simulink model "atrias_on_boom"  (R2018b)
settings: Solver=ode15s  StartTime=0.0  StopTime=inf  FixedStep=sample_time  MaxStep=1e-2  RelTol=1e-3
InitFcn:
  | addpath('../common/')
  | colors
  | simulation_params
  | mechanical_params
StartFcn:
  | clc
  | tic
StopFcn:
  | stopscript
values from neighbouring files (symbols this model uses):
  sample_time = 1/sample_freq    (= 0.001)    [simulation_params.m]
undefined symbols (not defined in the file or in its folder): Force_Control, rad, s, sgn, sm, t_friction, X, Y, Z
libraries: sm_lib x205, nesl_utility x123, simulink x49, fl_lib x16, mblibv1 x4, simulink_extras x2, powerlib_meascontrol x1
(part 8 of 8)

== system atrias_on_boom/Mechanical System Layer/R Leg/Thigh SEA/Rotor and Gearing ==
  Rotor Torque [Nm] : Inport
  Spring Torque [Nm] : Inport  Port=2
  Aligned Gear Constraint : sm_lib/Gears and Couplings/Gears/Common Gear Constraint  GearType=External  SpecificationType=CenterDistanceRatio  CenterDistance=(sm.r_rotor+sm.r_virtual_gear)/2  CenterDistanceUnits=m  GearRatio=1  BaseGearRadius=1  BaseGearRadiusUnits=m  FollGearRadius=1  FollGearRadiusUnits=m  AssemblyGearRotation=Free
      settings: SourceProductName=Simscape Multibody  SourceProductBaseCode=MS
  External Force and Torque : sm_lib/Forces and Torques/External Force and Torque  ForceResolutionFrame=AttachedFrame  EnableForceX=off  EnableForceY=off  EnableForceZ=off  EnableForce=off  TorqueResolutionFrame=AttachedFrame  EnableTorqueX=off  EnableTorqueY=off  EnableTorqueZ=on  EnableTorque=off
  Gear Offset : sm_lib/Frames and Transforms/Rigid Transform  TranslationMethod=Cartesian  TranslationStandardOffset=0  TranslationLengthUnit=m  TranslationStandardAxis=+Z  TranslationCartesianOffset=[(sm.r_rotor+sm.r_virtual_gear) 0 0]  TranslationROffset=0  TranslationROffsetUnits=m  TranslationZOffset=0  TranslationZOffsetUnits=m  TranslationThetaOffset=0  TranslationThetaOffsetUnits=deg  RotationMethod=None  RotationAngleUnits=deg  RotationStandardAxis=+Z  RotationAngle=0  RotationArbitraryAxis=[0 0 1]  FollAlignAxisA=+X  BaseAlignAxisA=+Y  FollAlignAxisB=+Y  BaseAlignAxisB=+Z  RotationSequenceAxes=FollowerAxes  RotationSequence=XYX  RotationSequenceAngles=[0 0 0]  RotationSequenceAnglesUnits=deg  RotationMatrix=[1 0 0; 0 1 0; 0 0 1]
  Idler Gear : sm_lib/Body Elements/Solid  InertiaType=Custom  Mass=sm.m_virtual_gear  MassUnits=kg  CenterOfMass=[0 0 0]  CenterOfMassUnits=m  MomentsOfInertia=sm.i_virtual_gear  MomentsOfInertiaUnits=kg*m^2  ProductsOfInertia=[0 0 0]  ProductsOfInertiaUnits=kg*m^2  BasedOnType=Density  Density=1000  DensityUnits=kg/(m^3)  DoExposeReferenceFrame=on  SerializedFrames=<Frames/>  GraphicType=None  MarkerShape=Sphere  MarkerSize=10  MarkerSizeUnits=m  GraphicVisPropType=SimpleVisualProperties  GraphicDiffuseColor=[1.0 0.2 0.2]  GraphicSpecularColor=[0.5 0.5 0.5 1.0]  GraphicAmbientColor=[0.15 0.15 0.15 1.0]  GraphicEmissiveColor=[0.0 0.0 0.0 1.0]  GraphicShininess=75  GraphicOpacity=1.0  GeometryShape=Cylinder  RectangleSize=[1 1]  RectangleSizeUnits=m  BrickDimensions=[1 1 1]  BrickDimensionUnits=m  CylinderRadius=sm.r_virtual_gear  CylinderRadiusUnits=m  CylinderLength=0.01  CylinderLengthUnits=m  SphereRadius=1  SphereRadiusUnits=m  EllipsoidRadii=[1 1 1]  EllipsoidRadiiUnits=m  ExtrusionCrossSection=[1 1; -1 1; -1 -1; 1 -1]  ExtrusionCrossSectionUnits=m  ExtrusionLength=.2  ExtrusionLengthUnits=m  PolygonNumSides=3  PolygonOuterRadius=.3  PolygonOuterRadiusUnits=m  ExtGeomFileType=STL  ExtGeomFileUnits=m  RevolutionCrossSection=[1 1; 1 -1; 2 -1; 2 1]  RevolutionCrossSectionUnits=m  RevolutionExtent=Full  RevolutionAngle=180  RevolutionAngleUnits=deg
  Idler Gear Constraint : sm_lib/Gears and Couplings/Gears/Common Gear Constraint  GearType=External  SpecificationType=CenterDistanceRatio  CenterDistance=(sm.r_rotor+sm.r_virtual_gear)/2  CenterDistanceUnits=m  GearRatio=1.0  BaseGearRadius=1  BaseGearRadiusUnits=m  FollGearRadius=1  FollGearRadiusUnits=m  AssemblyGearRotation=Free
      settings: SourceProductName=Simscape Multibody  SourceProductBaseCode=MS
  Idler Offset : sm_lib/Frames and Transforms/Rigid Transform  TranslationMethod=Cartesian  TranslationStandardOffset=0  TranslationLengthUnit=m  TranslationStandardAxis=+Z  TranslationCartesianOffset=[(sm.r_rotor+sm.r_virtual_gear)/2 0 0]  TranslationROffset=0  TranslationROffsetUnits=m  TranslationZOffset=0  TranslationZOffsetUnits=m  TranslationThetaOffset=0  TranslationThetaOffsetUnits=deg  RotationMethod=None  RotationAngleUnits=deg  RotationStandardAxis=+Z  RotationAngle=0  RotationArbitraryAxis=[0 0 1]  FollAlignAxisA=+X  BaseAlignAxisA=+Y  FollAlignAxisB=+Y  BaseAlignAxisB=+Z  RotationSequenceAxes=FollowerAxes  RotationSequence=XYX  RotationSequenceAngles=[0 0 0]  RotationSequenceAnglesUnits=deg  RotationMatrix=[1 0 0; 0 1 0; 0 0 1]
  Mechanical Rotational Reference : fl_lib/Mechanical/Rotational Elements/Mechanical Rotational Reference
  Opposite : Gain  Gain=-1
  Output Gear Joint : sm_lib/Joints/Revolute Joint  SenseConstraintForce=off  SenseConstraintForceX=off  SenseConstraintForceY=off  SenseConstraintForceZ=off  SenseConstraintTorque=off  SenseConstraintTorqueX=off  SenseConstraintTorqueY=off  SenseConstraintTorqueZ=off  SenseTotalForce=off  SenseTotalForceX=off  SenseTotalForceY=off  SenseTotalForceZ=off  SenseTotalTorque=off  SenseTotalTorqueX=off  SenseTotalTorqueY=off  SenseTotalTorqueZ=off  CompositeWrenchDir=FollowerOnBase  CompositeWrenchFrame=BaseFrame  EquilibriumPosition=0  EquilibriumPositionUnits=deg  SpringStiffness=0  SpringStiffnessUnits=N*m/deg  DampingCoefficient=0  DampingCoefficientUnits=N*m/(deg/s)  TorqueActuationMode=NoTorque  MotionActuationMode=ComputedMotion  SensePosition=on  SenseVelocity=on  SenseAcceleration=off  SenseTorqueForce=off  PositionTargetSpecify=off  PositionTargetPriority=High  PositionTargetValue=0  PositionTargetValueUnits=deg  VelocityTargetSpecify=off  VelocityTargetPriority=High  VelocityTargetValue=0  VelocityTargetValueUnits=deg/s
  Output Gear : sm_lib/Body Elements/Solid  InertiaType=Custom  Mass=sm.m_output_gear  MassUnits=kg  CenterOfMass=[0 0 0]  CenterOfMassUnits=m  MomentsOfInertia=sm.i_output_gear  MomentsOfInertiaUnits=kg*m^2  ProductsOfInertia=[0 0 0]  ProductsOfInertiaUnits=kg*m^2  BasedOnType=Density  Density=1000  DensityUnits=kg/(m^3)  DoExposeReferenceFrame=on  SerializedFrames=<Frames/>  GraphicType=None  MarkerShape=Sphere  MarkerSize=10  MarkerSizeUnits=m  GraphicVisPropType=SimpleVisualProperties  GraphicDiffuseColor=[1.0 0.2 0.0]  GraphicSpecularColor=[0.5 0.5 0.5 1.0]  GraphicAmbientColor=[0.15 0.15 0.15 1.0]  GraphicEmissiveColor=[0.0 0.0 0.0 1.0]  GraphicShininess=75  GraphicOpacity=1.0  GeometryShape=Cylinder  RectangleSize=[1 1]  RectangleSizeUnits=m  BrickDimensions=[1 1 1]  BrickDimensionUnits=m  CylinderRadius=0.03  CylinderRadiusUnits=m  CylinderLength=0.01  CylinderLengthUnits=m  SphereRadius=1  SphereRadiusUnits=m  EllipsoidRadii=[1 1 1]  EllipsoidRadiiUnits=m  ExtrusionCrossSection=[1 1; -1 1; -1 -1; 1 -1]  ExtrusionCrossSectionUnits=m  ExtrusionLength=1  ExtrusionLengthUnits=m  PolygonNumSides=3  PolygonOuterRadius=1  PolygonOuterRadiusUnits=m  ExtGeomFileType=STL  ExtGeomFileUnits=m  RevolutionCrossSection=[1 1; 1 -1; 2 -1; 2 1]  RevolutionCrossSectionUnits=m  RevolutionExtent=Full  RevolutionAngle=180  RevolutionAngleUnits=deg
  PS-Simulink Converter{,1..3} (4 alike) : nesl_utility/PS-Simulink Converter  PhysicalDomain=network_engine_domain  SubClassName=ps_output  LeftPortType=input  RightPortType=output  PseudoPeriodic=off  Frequencies=[]  Unit=1  AffineConversion=off
  Rotational Simscape Intf : Subsystem
  Rotational Friction : fl_lib/Mechanical/Rotational Elements/Rotational Friction  brkwy_trq=sm.breakaway_friction(2)/sm.N N*m  brkwy_vel=exp(-( (sm.friction_linear_zone(2)*sm.N) * 1 * (10) * 1 + 1/2) ) * ( (sm.friction_linear_zone(2)*sm.N) * 1 / 2 + 1 / ( (10) * 1) ) rad/s  Col_trq=sm.coulomb_friction(2)/sm.N N*m  visc_coef=sm.viscous_friction(2)/sm.N N*m/(rad/s)  w_specify=off  w_priority=High  w=0 rad/s  w_nominal_specify=off  w_nominal_unit=rad/s  w_nominal_value=1  t_specify=off  t_priority=High  t=0 N*m  t_nominal_specify=off  t_nominal_unit=N*m  t_nominal_value=1
      settings: SourceProductName=Simscape
  Rotor + Base Gear : sm_lib/Body Elements/Solid  InertiaType=Custom  Mass=sm.m_rotor  MassUnits=kg  CenterOfMass=[0 0 0]  CenterOfMassUnits=m  MomentsOfInertia=sm.i_rotor_moments  MomentsOfInertiaUnits=kg*m^2  ProductsOfInertia=[0 0 0]  ProductsOfInertiaUnits=kg*m^2  BasedOnType=Density  Density=1000  DensityUnits=kg/(m^3)  DoExposeReferenceFrame=on  SerializedFrames=<Frames/>  GraphicType=None  MarkerShape=Sphere  MarkerSize=10  MarkerSizeUnits=m  GraphicVisPropType=AdvancedVisualProperties  GraphicDiffuseColor=[0.5 0.5 0.5]  GraphicSpecularColor=[0.5 0.5 0.5 1.0]  GraphicAmbientColor=[0.15 0.15 0.15 1.0]  GraphicEmissiveColor=[0.0 0.0 0.0 1.0]  GraphicShininess=10  GraphicOpacity=1.0  GeometryShape=Cylinder  RectangleSize=[1 1]  RectangleSizeUnits=m  BrickDimensions=[1 1 1]  BrickDimensionUnits=m  CylinderRadius=0.01  CylinderRadiusUnits=m  CylinderLength=0.01  CylinderLengthUnits=m  SphereRadius=1  SphereRadiusUnits=m  EllipsoidRadii=[1 1 1]  EllipsoidRadiiUnits=m  ExtrusionCrossSection=[1 1; -1 1; -1 -1; 1 -1]  ExtrusionCrossSectionUnits=m  ExtrusionLength=0.4  ExtrusionLengthUnits=m  PolygonNumSides=3  PolygonOuterRadius=0.2  PolygonOuterRadiusUnits=m  ExtGeomFileType=STL  ExtGeomFileUnits=m  RevolutionCrossSection=[1 1; 1 -1; 2 -1; 2 1]  RevolutionCrossSectionUnits=m  RevolutionExtent=Full  RevolutionAngle=180  RevolutionAngleUnits=deg
  Rotor Joint : sm_lib/Joints/Revolute Joint  SenseConstraintForce=off  SenseConstraintForceX=off  SenseConstraintForceY=off  SenseConstraintForceZ=off  SenseConstraintTorque=off  SenseConstraintTorqueX=off  SenseConstraintTorqueY=off  SenseConstraintTorqueZ=off  SenseTotalForce=off  SenseTotalForceX=off  SenseTotalForceY=off  SenseTotalForceZ=off  SenseTotalTorque=off  SenseTotalTorqueX=off  SenseTotalTorqueY=off  SenseTotalTorqueZ=off  CompositeWrenchDir=FollowerOnBase  CompositeWrenchFrame=BaseFrame  EquilibriumPosition=0  EquilibriumPositionUnits=deg  SpringStiffness=0  SpringStiffnessUnits=N*m/deg  DampingCoefficient=0  DampingCoefficientUnits=N*m/(deg/s)  TorqueActuationMode=InputTorque  MotionActuationMode=ComputedMotion  SensePosition=off  SenseVelocity=on  SenseAcceleration=off  SenseTorqueForce=off  PositionTargetSpecify=off  PositionTargetPriority=High  PositionTargetValue=0  PositionTargetValueUnits=deg  VelocityTargetSpecify=off  VelocityTargetPriority=High  VelocityTargetValue=0  VelocityTargetValueUnits=deg/s
  Simulink-PS Converter : nesl_utility/Simulink-PS Converter  PhysicalDomain=network_engine_domain  SubClassName=ps_input  LeftPortType=input  RightPortType=output  PseudoPeriodic=off  Frequencies=[]  NoiseDistribution=none  NoiseParameters=[]  Unit=1  AffineConversion=off  FilteringAndDerivatives=zero  SimscapeFilterOrder=1  InputFilterTimeConstant=0.001  UdotUserProvided=1
  Simulink-PS Converter1 : nesl_utility/Simulink-PS Converter  PhysicalDomain=network_engine_domain  SubClassName=ps_input  LeftPortType=input  RightPortType=output  PseudoPeriodic=off  Frequencies=[]  NoiseDistribution=none  NoiseParameters=[]  Unit=1  AffineConversion=off  FilteringAndDerivatives=zero  SimscapeFilterOrder=1  InputFilterTimeConstant=0.001  UdotUserProvided=1
  Sum : Sum  Inputs=|++
  Virtual Gear Joint : sm_lib/Joints/Revolute Joint  SenseConstraintForce=off  SenseConstraintForceX=off  SenseConstraintForceY=off  SenseConstraintForceZ=off  SenseConstraintTorque=off  SenseConstraintTorqueX=off  SenseConstraintTorqueY=off  SenseConstraintTorqueZ=off  SenseTotalForce=off  SenseTotalForceX=off  SenseTotalForceY=off  SenseTotalForceZ=off  SenseTotalTorque=off  SenseTotalTorqueX=off  SenseTotalTorqueY=off  SenseTotalTorqueZ=off  CompositeWrenchDir=FollowerOnBase  CompositeWrenchFrame=BaseFrame  EquilibriumPosition=0  EquilibriumPositionUnits=deg  SpringStiffness=0  SpringStiffnessUnits=N*m/deg  DampingCoefficient=0  DampingCoefficientUnits=N*m/(deg/s)  TorqueActuationMode=NoTorque  MotionActuationMode=ComputedMotion  SensePosition=off  SenseVelocity=off  SenseAcceleration=off  SenseTorqueForce=off  PositionTargetSpecify=off  PositionTargetPriority=High  PositionTargetValue=0  PositionTargetValueUnits=deg  VelocityTargetSpecify=off  VelocityTargetPriority=High  VelocityTargetValue=0  VelocityTargetValueUnits=deg/s
  Virtual Follower Gear : sm_lib/Body Elements/Solid  InertiaType=Custom  Mass=sm.m_virtual_gear  MassUnits=kg  CenterOfMass=[0 0 0]  CenterOfMassUnits=m  MomentsOfInertia=sm.i_virtual_gear  MomentsOfInertiaUnits=kg*m^2  ProductsOfInertia=[0 0 0]  ProductsOfInertiaUnits=kg*m^2  BasedOnType=Density  Density=1000  DensityUnits=kg/(m^3)  DoExposeReferenceFrame=on  SerializedFrames=<Frames/>  GraphicType=None  MarkerShape=Sphere  MarkerSize=10  MarkerSizeUnits=m  GraphicVisPropType=SimpleVisualProperties  GraphicDiffuseColor=[1.0 0.2 0.2]  GraphicSpecularColor=[0.5 0.5 0.5 1.0]  GraphicAmbientColor=[0.15 0.15 0.15 1.0]  GraphicEmissiveColor=[0.0 0.0 0.0 1.0]  GraphicShininess=75  GraphicOpacity=1.0  GeometryShape=Cylinder  RectangleSize=[1 1]  RectangleSizeUnits=m  BrickDimensions=[1 1 1]  BrickDimensionUnits=m  CylinderRadius=sm.r_virtual_gear  CylinderRadiusUnits=m  CylinderLength=0.01  CylinderLengthUnits=m  SphereRadius=1  SphereRadiusUnits=m  EllipsoidRadii=[1 1 1]  EllipsoidRadiiUnits=m  ExtrusionCrossSection=[1 1; -1 1; -1 -1; 1 -1]  ExtrusionCrossSectionUnits=m  ExtrusionLength=.2  ExtrusionLengthUnits=m  PolygonNumSides=3  PolygonOuterRadius=.3  PolygonOuterRadiusUnits=m  ExtGeomFileType=STL  ExtGeomFileUnits=m  RevolutionCrossSection=[1 1; 1 -1; 2 -1; 2 1]  RevolutionCrossSectionUnits=m  RevolutionExtent=Full  RevolutionAngle=180  RevolutionAngleUnits=deg
  Virtual Gear Constraint : sm_lib/Gears and Couplings/Gears/Common Gear Constraint  GearType=External  SpecificationType=PitchCircleRadii  CenterDistance=20.0  CenterDistanceUnits=cm  GearRatio=1.0  BaseGearRadius=sm.r_rotor  BaseGearRadiusUnits=m  FollGearRadius=sm.r_virtual_gear  FollGearRadiusUnits=m  AssemblyGearRotation=Free
      settings: SourceProductName=Simscape Multibody  SourceProductBaseCode=MS
  Virtual Idler : sm_lib/Joints/Revolute Joint  SenseConstraintForce=off  SenseConstraintForceX=off  SenseConstraintForceY=off  SenseConstraintForceZ=off  SenseConstraintTorque=off  SenseConstraintTorqueX=off  SenseConstraintTorqueY=off  SenseConstraintTorqueZ=off  SenseTotalForce=off  SenseTotalForceX=off  SenseTotalForceY=off  SenseTotalForceZ=off  SenseTotalTorque=off  SenseTotalTorqueX=off  SenseTotalTorqueY=off  SenseTotalTorqueZ=off  CompositeWrenchDir=FollowerOnBase  CompositeWrenchFrame=BaseFrame  EquilibriumPosition=0  EquilibriumPositionUnits=deg  SpringStiffness=0  SpringStiffnessUnits=N*m/deg  DampingCoefficient=0  DampingCoefficientUnits=N*m/(deg/s)  TorqueActuationMode=NoTorque  MotionActuationMode=ComputedMotion  SensePosition=off  SenseVelocity=off  SenseAcceleration=off  SenseTorqueForce=off  PositionTargetSpecify=off  PositionTargetPriority=High  PositionTargetValue=0  PositionTargetValueUnits=deg  VelocityTargetSpecify=off  VelocityTargetPriority=High  VelocityTargetValue=0  VelocityTargetValueUnits=deg/s
  Rotor Conn : PMIOPort  Side=Left
  Gearhead Position [rad] : Outport
  Gearhead Velocity [rad/s] : Outport  Port=2
  Rotor Velocity [rad/s] : Outport  Port=3
  wires:
  PS-Simulink Converter1/1 -> Gearhead Position [rad]/1
  Rotor Torque [Nm]/1 -> Sum/1
  PS-Simulink Converter2/1 -> Gearhead Velocity [rad/s]/1
  PS-Simulink Converter3/1 -> Rotor Velocity [rad/s]/1
  Spring Torque [Nm]/1 -> Opposite/1
  Opposite/1 -> Simulink-PS Converter1/1
  Sum/1 -> Simulink-PS Converter/1
  PS-Simulink Converter/1 -> Sum/2
  connections:
  Virtual Gear Joint/RConn1 -- Virtual Follower Gear/RConn1 -- Virtual Gear Constraint/RConn1 -- Idler Gear Constraint/LConn1
  External Force and Torque/RConn1 -- Output Gear/RConn1 -- Aligned Gear Constraint/RConn1 -- Output Gear Joint/RConn1
  Gear Offset/RConn1 -- Virtual Gear Joint/LConn1
  Gear Offset/LConn1 -- Rotor Joint/LConn1 -- Rotor Conn/RConn1 -- Output Gear Joint/LConn1 -- Idler Offset/LConn1
  Rotor Joint/RConn1 -- Virtual Gear Constraint/LConn1 -- Rotor + Base Gear/RConn1
  Simulink-PS Converter/RConn1 -- Rotor Joint/LConn2
  PS-Simulink Converter2/LConn1 -- Output Gear Joint/RConn3
  PS-Simulink Converter1/LConn1 -- Output Gear Joint/RConn2
  PS-Simulink Converter3/LConn1 -- Rotational Simscape Intf/LConn1 -- Rotor Joint/RConn2
  Simulink-PS Converter1/RConn1 -- External Force and Torque/LConn1
  Idler Gear Constraint/RConn1 -- Virtual Idler/RConn1 -- Idler Gear/RConn1 -- Aligned Gear Constraint/LConn1
  Idler Offset/RConn1 -- Virtual Idler/LConn1
  PS-Simulink Converter/LConn1 -- Rotational Simscape Intf/RConn1
  Rotational Friction/RConn1 -- Mechanical Rotational Reference/LConn1 -- Rotational Simscape Intf/RConn2
  Rotational Friction/LConn1 -- Rotational Simscape Intf/LConn2

== system atrias_on_boom/Mechanical System Layer/Right Hip Roll Joint/Mechanical Limits /Enabled Subsystem ==
  Col_Flags : Inport
  Enable : EnablePort  StatesWhenEnabling=reset  ZeroCross=off
  To Workspace : ToWorkspace  VariableName=R_roll_collision_flags  SampleTime=-1
  wires:
  Col_Flags/1 -> To Workspace/1

== system atrias_on_boom/Mechanical System Layer/Right Hip Roll Joint/Mechanical Limits /Roll Max Collision Model ==
  note: Mechanical Limits Model
  phi [rad] : Inport
  vphi [rad/s] : Inport  Port=2
  Contact! : EnablePort  StatesWhenEnabling=reset
  Gain3 : Gain  Gain=sm.k_phi
  Gain4 : Gain  Gain=1/sm.v_phi_max
  Mux1 : Mux  Inputs=2
  Reaction Force : Fcn  Expr="- u(1)  *  (1-u(2)) * (u(2)<1)"
  tau_interaction[Nm] : Outport  OutputWhenDisabled=reset  InitialOutput=0
      settings: AttributesFormatString=initial = '%<InitialOutput>'\nwhen disabled = '%<OutputWhenDisabled>'
  wires:
  Gain4/1 -> Mux1/2
  Mux1/1 -> Reaction Force/1
  vphi [rad/s]/1 -> Gain4/1
  phi [rad]/1 -> Gain3/1
  Gain3/1 -> Mux1/1
  Reaction Force/1 -> tau_interaction[Nm]/1

== system atrias_on_boom/Mechanical System Layer/Right Hip Roll Joint/Mechanical Limits /Roll Min Collision Model ==
  note: Mechanical Limits Model
  phi [rad] : Inport
  vphi [rad/s] : Inport  Port=2
  Contact! : EnablePort  StatesWhenEnabling=reset
  Gain3 : Gain  Gain=sm.k_phi
  Gain4 : Gain  Gain=1/sm.v_phi_max
  Mux1 : Mux  Inputs=2
  Reaction Force : Fcn  Expr="- u(1)  *  (1-u(2)) * (u(2)<1)"
  tau_interaction[Nm] : Outport  OutputWhenDisabled=reset  InitialOutput=0
      settings: AttributesFormatString=initial = '%<InitialOutput>'\nwhen disabled = '%<OutputWhenDisabled>'
  wires:
  Gain3/1 -> Mux1/1
  phi [rad]/1 -> Gain3/1
  vphi [rad/s]/1 -> Gain4/1
  Mux1/1 -> Reaction Force/1
  Gain4/1 -> Mux1/2
  Reaction Force/1 -> tau_interaction[Nm]/1

== system atrias_on_boom/behavior_controller/Behavior/Leg Switch/Left Stance Timing ==
  Td : Inport
  System Time : Inport  Port=2
  Enable : EnablePort
  Memory : Memory
  Sum : Sum  Inputs=|+-
  Ts : Outport
  wires:
  System Time/1 -> Sum/1
  Td/1 -> Sum/2
  Memory/1 -> Ts/1
  Sum/1 -> Memory/1

== system atrias_on_boom/behavior_controller/Behavior/Leg Switch/Left Swing Timing ==
  System Time : Inport
  Enable : EnablePort
  Td : Outport
  wires:
  System Time/1 -> Td/1

== system atrias_on_boom/behavior_controller/Behavior/Leg Switch/Right Stance Timing ==
  System Time : Inport
  Td : Inport  Port=2
  Enable : EnablePort
  Memory : Memory
  Sum : Sum  Inputs=|+-
  Ts : Outport
  wires:
  System Time/1 -> Sum/1
  Td/1 -> Sum/2
  Memory/1 -> Ts/1
  Sum/1 -> Memory/1

== system atrias_on_boom/behavior_controller/Behavior/Leg Switch/Right Swing Timing ==
  System Time : Inport
  Enable : EnablePort
  Td : Outport
  wires:
  System Time/1 -> Td/1

== system atrias_on_boom/behavior_controller/Behavior/Leg Switch/dxTO for LLeg control ==
  vx_torso : Inport
  Enable : EnablePort
  dxTO : Outport
  wires:
  vx_torso/1 -> dxTO/1

== system atrias_on_boom/behavior_controller/Behavior/Leg Switch/dxTO for RLeg control ==
  vx_torso : Inport
  Enable : EnablePort
  dxTO : Outport
  wires:
  vx_torso/1 -> dxTO/1

== system atrias_on_boom/behavior_controller/Behavior/Swing Leg Control/Swing Trajectory ==
  thetas : Inport
  theta_dots : Inport  Port=2
  Ts : Inport  Port=3
  vx_torso : Inport  Port=4
  "[x,z]_torso" : Inport  Port=5
  leg_lengths : Inport  Port=6
  Time : Inport  Port=7
  Enable : EnablePort  PropagateVarSize=During execution
  " " : Constant  Value=0
  " 1" : Constant  Value=0
  " 2" : Constant  Value=sm.v_avg
  Constant : Constant  Value=100
  Constant1 : Constant  Value=0.2
  Five-bar Diff FK (approx) : MATLAB Function  TreatAsAtomicUnit=on
  Five-bar FK : MATLAB Function  TreatAsAtomicUnit=on
  Mux1 : Mux  Inputs=2
  Mux2 : Mux
  Mux4 : Mux
  Sum : Sum  Inputs=++|
  Sum1 : Sum  Inputs=++|
  Swing Trajectory Fit : MATLAB Function  TreatAsAtomicUnit=on  SystemSampleTime=0.005
  desired foot placement wrt COM : Fcn  Expr=u(2)*u(1)/2 - sm.Kv * (sm.v_avg-u(1))
  Trajectory : Outport
  Origin : Outport  Port=2
  Td : Outport  Port=3
  wires:
  Swing Trajectory Fit/1(trajectory) -> Trajectory/1
  Ts/1 -> Swing Trajectory Fit/4(Ts), Mux1/2
  Constant/1 -> Swing Trajectory Fit/5(num_points)
  Constant1/1 -> Swing Trajectory Fit/3(clearance)
  Mux1/1 -> desired foot placement wrt COM/1
  vx_torso/1 -> Mux1/1
  desired foot placement wrt COM/1 -> Sum/2  "x_offset"
  " "/1 -> Sum1/2  "z_offset"
  "[x,z]_torso"/1 -> Origin/1
  Five-bar FK/1(x) -> Sum/1, Mux2/1
  Five-bar FK/2(z) -> Sum1/1, Mux2/2
  Mux2/1 -> Swing Trajectory Fit/1(pos_init)
  leg_lengths/1 -> Five-bar Diff FK (approx)/1(lengths), Five-bar FK/1(lengths)
  Time/1 -> Td/1
  thetas/1 -> Five-bar Diff FK (approx)/2(thetas), Five-bar FK/2(thetas)
  Five-bar Diff FK (approx)/1(x_dot) -> Mux2/3
  Five-bar Diff FK (approx)/2(z_dot) -> Mux2/4
  Sum/1 -> Mux4/1  "x_end"
  Sum1/1 -> Mux4/2  "z_end"
  Mux4/1 -> Swing Trajectory Fit/2(pos_end)
  " 1"/1 -> Mux4/4  "vz_end"
  " 2"/1 -> Mux4/3  "vx_end"
  theta_dots/1 -> Five-bar Diff FK (approx)/3(theta_dots)

== system atrias_on_boom/Mechanical System Layer/L Ground Contact/Ground Friction Model/t-Axis Kinetic Friction Model/Magnitude ==
  Vector : Inport
  Sqrt : Sqrt  OutputSignalType=real  SaturateOnIntegerOverflow=on
  Square : Math  Operator=square  OutputSignalType=real  SaturateOnIntegerOverflow=on
  Sum of Elements : Sum  Inputs=+
  Magnitude : Outport
  wires:
  Vector/1 -> Square/1
  Sum of Elements/1 -> Sqrt/1
  Square/1 -> Sum of Elements/1
  Sqrt/1 -> Magnitude/1

== system atrias_on_boom/Mechanical System Layer/L Ground Contact/Ground Friction Model/t-Axis Static Friction Model/Magnitude ==
  Vector : Inport
  Sqrt : Sqrt  OutputSignalType=real  SaturateOnIntegerOverflow=on
  Square : Math  Operator=square  OutputSignalType=real  SaturateOnIntegerOverflow=on
  Sum of Elements : Sum  Inputs=+
  Magnitude : Outport
  wires:
  Vector/1 -> Square/1
  Sum of Elements/1 -> Sqrt/1
  Square/1 -> Sum of Elements/1
  Sqrt/1 -> Magnitude/1

== system atrias_on_boom/Mechanical System Layer/L Leg/Shin SEA/Rotor and Gearing/Rotational Simscape Intf ==
  Ideal Angular Velocity Source : fl_lib/Mechanical/Mechanical Sources/Ideal Angular Velocity Source
  Ideal Torque Sensor : fl_lib/Mechanical/Mechanical Sensors/Ideal Torque Sensor
  w : PMIOPort  Side=Left
  T : PMIOPort  Port=2  Side=Right
  R : PMIOPort  Port=3  Side=Left
  C : PMIOPort  Port=4  Side=Right
  connections:
  w/RConn1 -- Ideal Angular Velocity Source/RConn1
  T/RConn1 -- Ideal Torque Sensor/RConn2
  Ideal Torque Sensor/LConn1 -- Ideal Angular Velocity Source/RConn2
  R/RConn1 -- Ideal Angular Velocity Source/LConn1
  Ideal Torque Sensor/RConn1 -- C/RConn1

== system atrias_on_boom/Mechanical System Layer/L Leg/Thigh SEA/Rotor and Gearing/Rotational Simscape Intf ==
  Ideal Angular Velocity Source : fl_lib/Mechanical/Mechanical Sources/Ideal Angular Velocity Source
  Ideal Torque Sensor : fl_lib/Mechanical/Mechanical Sensors/Ideal Torque Sensor
  w : PMIOPort  Side=Left
  T : PMIOPort  Port=2  Side=Right
  R : PMIOPort  Port=3  Side=Left
  C : PMIOPort  Port=4  Side=Right
  connections:
  w/RConn1 -- Ideal Angular Velocity Source/RConn1
  T/RConn1 -- Ideal Torque Sensor/RConn2
  Ideal Torque Sensor/LConn1 -- Ideal Angular Velocity Source/RConn2
  R/RConn1 -- Ideal Angular Velocity Source/LConn1
  Ideal Torque Sensor/RConn1 -- C/RConn1

== system atrias_on_boom/Mechanical System Layer/R Ground Contact/Ground Friction Model/t-Axis Kinetic Friction Model/Magnitude ==
  Vector : Inport
  Sqrt : Sqrt  OutputSignalType=real  SaturateOnIntegerOverflow=on
  Square : Math  Operator=square  OutputSignalType=real  SaturateOnIntegerOverflow=on
  Sum of Elements : Sum  Inputs=+
  Magnitude : Outport
  wires:
  Sqrt/1 -> Magnitude/1
  Square/1 -> Sum of Elements/1
  Sum of Elements/1 -> Sqrt/1
  Vector/1 -> Square/1

== system atrias_on_boom/Mechanical System Layer/R Ground Contact/Ground Friction Model/t-Axis Static Friction Model/Magnitude ==
  Vector : Inport
  Sqrt : Sqrt  OutputSignalType=real  SaturateOnIntegerOverflow=on
  Square : Math  Operator=square  OutputSignalType=real  SaturateOnIntegerOverflow=on
  Sum of Elements : Sum  Inputs=+
  Magnitude : Outport
  wires:
  Sqrt/1 -> Magnitude/1
  Square/1 -> Sum of Elements/1
  Sum of Elements/1 -> Sqrt/1
  Vector/1 -> Square/1

== system atrias_on_boom/Mechanical System Layer/R Leg/Shin SEA/Rotor and Gearing/Rotational Simscape Intf ==
  Ideal Angular Velocity Source : fl_lib/Mechanical/Mechanical Sources/Ideal Angular Velocity Source
  Ideal Torque Sensor : fl_lib/Mechanical/Mechanical Sensors/Ideal Torque Sensor
  w : PMIOPort  Side=Left
  T : PMIOPort  Port=2  Side=Right
  R : PMIOPort  Port=3  Side=Left
  C : PMIOPort  Port=4  Side=Right
  connections:
  Ideal Torque Sensor/RConn1 -- C/RConn1
  R/RConn1 -- Ideal Angular Velocity Source/LConn1
  Ideal Torque Sensor/LConn1 -- Ideal Angular Velocity Source/RConn2
  T/RConn1 -- Ideal Torque Sensor/RConn2
  w/RConn1 -- Ideal Angular Velocity Source/RConn1

== system atrias_on_boom/Mechanical System Layer/R Leg/Thigh SEA/Rotor and Gearing/Rotational Simscape Intf ==
  Ideal Angular Velocity Source : fl_lib/Mechanical/Mechanical Sources/Ideal Angular Velocity Source
  Ideal Torque Sensor : fl_lib/Mechanical/Mechanical Sensors/Ideal Torque Sensor
  w : PMIOPort  Side=Left
  T : PMIOPort  Port=2  Side=Right
  R : PMIOPort  Port=3  Side=Left
  C : PMIOPort  Port=4  Side=Right
  connections:
  Ideal Torque Sensor/RConn1 -- C/RConn1
  R/RConn1 -- Ideal Angular Velocity Source/LConn1
  Ideal Torque Sensor/LConn1 -- Ideal Angular Velocity Source/RConn2
  T/RConn1 -- Ideal Torque Sensor/RConn2
  w/RConn1 -- Ideal Angular Velocity Source/RConn1

== matlab function atrias_on_boom/Mechanical System Layer/L Ground Contact/determine_ground_height ==
  data: yaw input; zGround output; tile_width input; tile_scale input
function zGround = fcn(yaw, tile_width, tile_scale)
index = floor(yaw/tile_width)+1;
index = max(min(index, 12),1);
zGround = tile_scale(index);

== matlab function atrias_on_boom/Mechanical System Layer/Torso/Rotate Vector ==
  settings: updateMethod=DISCRETE
  data: R input; rotated output; v input
function rotated  = rotate_vector(R, v)  
    
  rotated = R'*v;
    
end

== matlab function atrias_on_boom/behavior_controller/Behavior/Swing Leg Control/Five-bar IK ==
  data: xz input; thetas output; lengths input
function thetas = fcn(xz,lengths)
    % thetas - [theta_b, theta_f] in range [0,2*pi]
    % lengths - [l_b_th, l_b_sh, l_f_th, l_f_sh, l_f_off]
    l1 = lengths(1); % l_b_th
    l2 = lengths(2); % l_b_sh
    l3 = lengths(3); % l_f_th
    l4 = lengths(4); % l_f_sh
    l5 = lengths(5); % l_f_off
    
    x = xz(1);
    z = xz(2);
    thetas = [0,0];
    theta_foot = atan2(z,x);
    if (theta_foot < 0)
        theta_foot = theta_foot + 2*pi;
    end
    d_foot = sqrt(x^2+z^2);
    thetas(2) = theta_foot + acos((d_foot^2 + l3^2 - (l4+l5)^2)/(2*d_foot*l3));
    
    theta_knee_f = pi + acos((l3^2 + (l4+l5)^2 - (x^2+z^2))/(2*l3*(l4+l5)));
    x_ankle = x - l5*cos(theta_knee_f + thetas(2));
    z_ankle = z - l5*sin(theta_knee_f + thetas(2));
    theta_ankle = atan2(z_ankle,x_ankle);
    if (theta_ankle < 0)
        theta_ankle = theta_ankle + 2*pi;
    end
    d_ankle = sqrt(x_ankle^2+z_ankle^2);
    thetas(1) = theta_ankle - acos((d_ankle^2 + l1^2 - l2^2)/(2*d_ankle*l1));
end

== matlab function atrias_on_boom/behavior_controller/Behavior/Swing Leg Control/Interpolate ==
  data: trajectory input; origin input; xz output; t input
function xz = fcn(trajectory, origin, t)
    if (t>trajectory(end,1))
        xz = trajectory(end,2:3);
    else
        xz = zeros(1,2);
        xz(1) = interp1(trajectory(:,1), trajectory(:,2), t);
        xz(2) = interp1(trajectory(:,1), trajectory(:,3), t);
    end
    xz(1) = xz(1) + origin(1);
    xz(2) = xz(2) + origin(2);
end

== matlab function atrias_on_boom/Mechanical System Layer/R Ground Contact/determine_ground_height ==
  data: yaw input; zGround output; tile_width input; tile_scale input
function zGround = fcn(yaw, tile_width, tile_scale)
index = floor(yaw/tile_width)+1;
index = max(min(index, 12),1);
zGround = tile_scale(index);

== matlab function atrias_on_boom/behavior_controller/Behavior/Swing Leg Control/Swing Trajectory/Five-bar Diff FK (approx) ==
  data: x_dot output; lengths input; z_dot output; thetas input; theta_dots input
function [x_dot,z_dot] = fcn(lengths, thetas, theta_dots)
    % theta - [theta_b, theta_f]
    % lengths - [l_b_th, l_b_sh, l_f_th, l_f_sh, l_f_off]
    l1 = lengths(1); % l_b_th
    l2 = lengths(2); % l_b_sh
    l3 = lengths(3); % l_f_th
    l4 = lengths(4); % l_f_sh
    l5 = lengths(5); % l_f_off
    
    assert(thetas(2) > thetas(1), sprintf('Front angle(%f) < Back angle(%f)',thetas(2),thetas(1)));
    
    l = 0.25*(l1+l2+l3+l4);
    
%     v_par = -l*sin((thetas(2) - thetas(1))/2)*(theta_dots(2) - theta_dots(1));
%     v_perp = l*cos((thetas(2) - thetas(1))/2)*(theta_dots(2) + theta_dots(1));
    
    x_dot = -l*theta_dots(1)*sin(thetas(1)) - l*theta_dots(2)*sin(thetas(2));
    z_dot = l*theta_dots(1)*cos(thetas(1)) + l*theta_dots(2)*cos(thetas(2));
    
end

== matlab function atrias_on_boom/behavior_controller/Behavior/Swing Leg Control/Swing Trajectory/Five-bar FK ==
  data: x output; lengths input; z output; thetas input
function [x,z] = fcn(lengths, thetas)
    % theta - [theta_b, theta_f]
    % lengths - [l_b_th, l_b_sh, l_f_th, l_f_sh, l_f_off]
    l1 = lengths(1); % l_b_th
    l2 = lengths(2); % l_b_sh
    l3 = lengths(3); % l_f_th
    l4 = lengths(4); % l_f_sh
    l5 = lengths(5); % l_f_off
    
    assert(thetas(2) > thetas(1), sprintf('Front angle(%f) < Back angle(%f)',thetas(2),thetas(1)));
    
    x_knee_b = l1*cos(thetas(1));
    z_knee_b = l1*sin(thetas(1));
    
    x_knee_f = l3*cos(thetas(2));
    z_knee_f = l3*sin(thetas(2));
    
    theta_hip = thetas(2) - thetas(1);
    theta_ankle = acos((l2^2 + l4^2 - ((x_knee_b-x_knee_f)^2 + (z_knee_b-z_knee_f)^2))/(2*l2*l4));
    
    % 2pi - theta_hip - theta_ankle = theta_knee_f + theta_knee_b
    % l_f_th^2 + l_f_sh^2 - 2(l_f_th)(l_f_sh)cos(theta_knee_f) = l_b_th^2 + l_b_sh^2 - 2(l_b_th)(l_b_sh)cos(theta_knee_b)
    c = 2*pi -theta_hip - theta_ankle;
    alpha = atan2(-l3*l4*sin(c),l1*l2-l3*l4*cos(c));
    if (alpha<0)
        alpha = 2*pi+alpha;
    end
    
    theta_1 = acos((l3^2 + l4^2 - l1^2 - l2^2)/(2*sqrt((l3*l4*sin(c))^2+(l1*l2-l3*l4*cos(c))^2)));
    theta_knee_f1 = alpha + theta_1;
    theta_knee_f2 = alpha - theta_1;
    
    if (theta_knee_f1 > 2*pi)
        theta_knee_f1 = theta_knee_f1 - 2*pi;
    end

    if (theta_knee_f2 < 0)
        theta_knee_f2 = theta_knee_f2 + 2*pi;
    end
    
    if ((theta_knee_f1 > 0) && ((c - theta_knee_f1) > 0))
        theta_knee_f = theta_knee_f1+pi;
    elseif((theta_knee_f2 > 0) && ((c - theta_knee_f2) > 0))
        theta_knee_f = theta_knee_f2+pi;
    else
        theta_knee_f = min(abs(theta_knee_f1), abs(theta_knee_f2));
    end
    
   x = x_knee_f + (l4+l5)*cos(theta_knee_f + thetas(2));
   z = z_knee_f + (l4+l5)*sin(theta_knee_f + thetas(2));
    
end

== matlab function atrias_on_boom/behavior_controller/Behavior/Swing Leg Control/Swing Trajectory/Swing Trajectory Fit ==
  data: pos_init input; trajectory output size=[100 3]; pos_end input; clearance input; Ts input; num_points input
function trajectory = fcn(pos_init, pos_end, clearance, Ts, num_points)
    
    t_points = [0,Ts/2,Ts];
    x_points = [pos_init(1), (pos_init(1) + pos_end(1))/2, pos_end(1)];
    z_points = [pos_init(2), clearance+(pos_init(2) + pos_end(2))/2, pos_end(2)];
    
    t_q = linspace(0,Ts,num_points);
%     x_spline = csape(t_points, x_points, 'complete', [pos_init(3), pos_end(3)]);
%     z_spline = csape(t_points, z_points, 'complete', [pos_init(4), pos_end(4)]);
    x_spline = spline(t_points, x_points, t_q);
    z_spline = spline(t_points, z_points, t_q);
    
%     trajectory = [t_q', fnval(x_spline, tq)', fnval(z_spline, tq)'];
    trajectory = [t_q', x_spline', z_spline'];
    
%     l_th_f = 0.5;
%     l_th_b = 0.5;
%     l_sh_f = 0.4;
%     l_sh_b = 0.4;
%     l_sh_off = 0.15;
%     for i=1:1:size(traj,1)
%         x = traj(i,1);
%         y = traj(i,2);
%         theta_th_f = acos(x/sqrt(x^2+y^2)) - acos((x^2 + y^2 + l_th_f^2 - (l_sh_f+l_sh_off)^2)/((2*l_th_f)*(sqrt(x^2+y^2))));
%     end
    
end

== matlab function atrias_on_boom/Mechanical System Layer/Torso/Rotation To Euler Angles ==
  settings: updateMethod=DISCRETE
  data: R input; roll output; pitch output; yaw output
function  [roll, pitch, yaw] = rotation_to_euler(R)  
    
    persistent curyaw
    if isempty(curyaw)
        curyaw = 0;
    end

    newyaw = atan2( R(2,1), R(1,1));
    pitch  = atan2(-R(3,1), sqrt(R(3,2)^2+R(3,3)^2));
    roll   = atan2( R(3,2), R(3,3));
    curyaw = curyaw + mod(newyaw - curyaw + pi, 2*pi) - pi;
    yaw = curyaw;
    
end

== matlab function atrias_on_boom/behavior_controller/Behavior/Convert to Body Frame IMU Accelerations ==
  data: accelerometer input; imu_accelerations output
function imu_accelerations = imu_to_body_frame(accelerometer)
    g = 9.803;
    z_up_rotation = [1, 0, 0; 0, 0, 1; 0, -1, 0];
    align_xy_rotation = [sqrt(2)/2, -sqrt(2)/2, 0; sqrt(2)/2, sqrt(2)/2, 0; 0, 0, 1];
    imu_accelerations = g*z_up_rotation*align_xy_rotation*accelerometer;
end
